simulink model "Experiment_134_cs"  (Simulink 10.1)
settings: Solver=ode8  StartTime=0.0  StopTime=20  FixedStep=1/10  RelTol=1e-3
model workspace (MAT data in the model file):
  mbox_table : struct (value not decoded)
  model_closed = 0
  sim_status = 0
PreLoadFcn:
  | mbxruntime.callbacks.PreLoadFcn(bdroot);
PostLoadFcn:
  | mbxruntime.callbacks.PostLoadFcn(bdroot);
InitFcn:
  | mbxruntime.callbacks.InitFcn(bdroot);
StartFcn:
  | mbxruntime.callbacks.StartFcn(bdroot);
StopFcn:
  | mbxruntime.callbacks.StopFcn(bdroot);
undefined symbols (not defined in the file or in its folder): acce_1, acce_2, acce_3, brake, steer, steer_1, steer_2, steer_3, t0_1, t0_2, t0_3, throttle, v_1, v_2, v_3, v_4
libraries: simulink x79, simulink_extras x12, PreScanSimulinkLibrary x8
(part 1 of 9)
CloseFcn:
  | mbxruntime.callbacks.CloseFcn(bdroot);
settings Model: Creator=PRESCAN  LastModifiedBy=Administrator
settings DataIOCC: LimitDataPoints=on  SignalLoggingSaveFormat=ModelDataLogs
settings OptimizationCC: ExpressionDepthLimit=2147483647  InitFltsAndDblsToZero=on
settings DebuggingCC: SaveWithParameterizedLinksMsg=none  SignalResolutionControl=TryResolveAllWithWarning  MultiTaskDSMMsg=warning  MultiTaskCondExecSysMsg=none  FcnCallInpInsideContextMsg=warning  StateNameClashWarn=warning
settings ModelReferenceCC: UpdateModelReferenceTargets=IfOutOfDate
settings SFSimCC: SimParseCustomCode=off
settings SFSimCC: SimCustomHeaderCode=|
  | #include "prescan.h"
  | #include "prescan_platform.h"
settings GRTTargetCC: TargetFcnLib=ansi_tfl_tmw.mat

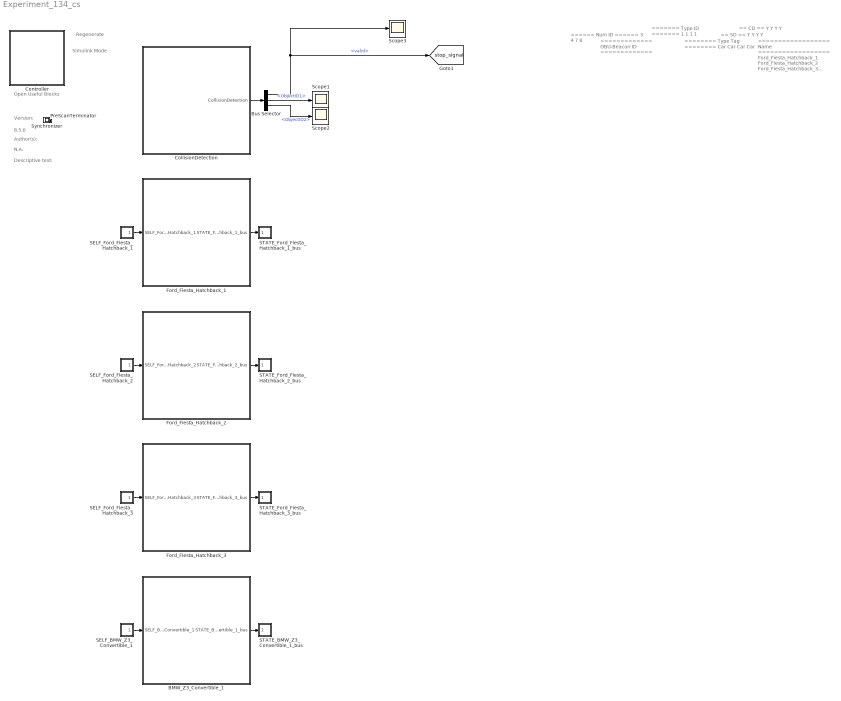
== system Experiment_134_cs ==
  note: Regenerate
  note: Simulink Mode
  note: Open Useful Blocks
  note: 8.5.0
  note: Version:
  note: Author(s):
  note: N.A.
  note: Descriptive text:
  note: ======
      | Num ID
      | ======
      | 3
      | 4
      | 7
      | 8
  note: =============
      | OBU-Beacon ID
      | =============
  note: =======
      | Type ID
      | =======
      | 1
      | 1
      | 1
      | 1
  note: ========
      | Type Tag
      | ========
      | Car
      | Car
      | Car
      | Car
  note: ==
      | SD
      | ==
      | Y
      | Y
      | Y
      | Y
  note: ==
      | CD
      | ==
      | Y
      | Y
      | Y
      | Y
  note: ==================
      | Name
      | ==================
      | Ford_Fiesta_Hatchback_1
      | Ford_Fiesta_Hatchback_2
      | Ford_Fiesta_Hatchback_3
      | BMW_Z3_Convertible_1
  BMW_Z3_Convertible_1 : Subsystem  Tag=WorldObjectSubSystem  InitFcn=UniqueId = '511';
      mask init:
      | modelPath = GenericModelHelper.getGenericModelFilePath('ModelDepo','Vehicles\BMW_Z3\BMW_Z3.pgmb','7699e47834166b94c09717861bab4f7a');imagePath = GenericModelHelper.getCompilationPicture(modelPath, 'BMW_Z3_HighPoly.png');
      mask Display: image(imread(imagePath));color('white');text(0, 0, ' ID=8\n')
  Bus Selector : BusSelector  OutputSignals=HEADER.valid,DATA.ObjectID1,DATA.ObjectID2
  CollisionDetection : Subsystem  Tag=sensor/CollisionDetection  Priority=1  LoadFcn=load('PrescanCollisionDetectionData.mat');load('PrescanCollisionDetectionMessage.mat')  mask(PreScan Source Block: CollisionDetection){}
      mask help: Collision Detection can be used to detect collisions between PreScan components. For Collision Detection the actual component shape is taken into account, so it is not a bounding box approach.
      settings: OpenFcn=open_system([gcb '/Sensor'],'mask')
      mask Help: eval('openHelp(811)')
      mask Display: image(imread('crash.jpg'))
  Controller : Subsystem  Description=648A510100055748DE7A0D51105FBAC79BDC343D1789F8D295123B632F6EF672  Priority=-1  LoadFcn=load PreScanControllerData  mask(PreScan Simulation Controller){prescanversion='8.5.0', ModelReferencing=off, TimeStep=1/10, ControlMode=0, PreScanExecutionMode=on, ControllerCount=0, ControllerIndex=0, ControllerOptions=''}
      mask prompts: prescanversion "PreScan Version"; ModelReferencing "Use Model Referencing"; TimeStep "Upload Period [s]"; ControlMode "Control Mode"; PreScanExecutionMode "Execution Mode"; ControllerCount "Controller Count"; ControllerIndex "Controller Index"; ControllerOptions "Controller Options"
      mask help:
      | Please do not remove this block from the compilation sheet,
      | as it connects the model to the PreScan environment.
      mask init:
      | model = bdroot(gcb);
      | ExperimentFile = mbxruntime.findExperimentFile(model,true); %relative path
      | 
      | [d1, d2, d3, prescandata] = prescan_Settings();
      | ModelDepo = fullfile(prescandata,'ModelDepo'); 
      | 
      | RTmode = mbxruntime.getRTMode(model);
      | 
      | SimulationMode = get_param(bdroot,'SimulationMode');
      | if strcmp(SimulationMode, 'rapid-accelerator')
      |     SimulationMode = 'external';
      | end
      | TargetName = get_param(bdroot,'SystemTargetFile');
      settings: ModelCloseFcn=assignin('base',['model_closed_' bdroot],true);
      mask Help: eval('openHelp(812)')
      mask Display: image(imread('prescanlogo.ico'))
  Ford_Fiesta_Hatchback_1 : Subsystem  Tag=WorldObjectSubSystem  InitFcn=UniqueId = '405';
      mask init:
      | modelPath = GenericModelHelper.getGenericModelFilePath('ModelDepo','Vehicles\Ford_Fiesta\Ford_Fiesta.pgmb','ee79ea2575daad9b4625620a37d79be4');imagePath = GenericModelHelper.getCompilationPicture(modelPath, 'Ford_Fiesta_HighPoly.png');
      mask Display: image(imread(imagePath));color('white');text(0, 0, ' ID=3\n')
  Ford_Fiesta_Hatchback_2 : Subsystem  Tag=WorldObjectSubSystem  InitFcn=UniqueId = '485';
      mask init: same as Experiment_134_cs/Ford_Fiesta_Hatchback_1
      mask Display: image(imread(imagePath));color('white');text(0, 0, ' ID=4\n')
  Ford_Fiesta_Hatchback_3 : Subsystem  Tag=WorldObjectSubSystem  InitFcn=UniqueId = '486';
      mask init: same as Experiment_134_cs/Ford_Fiesta_Hatchback_1
      mask Display: image(imread(imagePath));color('white');text(0, 0, ' ID=7\n')
  PreScanTerminator : Subsystem  Tag=PreScanTerminator  Priority=999  LoadFcn=load PrescanTerminatorData  mask(PreScan Simulation Terminator){TimeStep=1/10}
      mask prompts: TimeStep "Upload Period [s]"
      mask help:
      | Please do not remove this block from the compilation sheet as it
      | connects the model to the PreScan environment.
      mask Help: eval('openHelp(812)')
      mask Display: image(imread('prescanlogo.ico'))
  SELF_BMW_Z3_Convertible_1 : Subsystem  Tag=sensor/SelfPort  Priority=1  LoadFcn=load('PreScanSelfSensorData.mat')  mask(PreScan Source Block: SELF){}
      mask help:
      | The SELF port shows (state) information of the actor itself. The outputs are position in the experiment's axis system and the GPS coordinates, and the object's absolute velocity and compass heading.
      |
      | For more information, please click Help.
      settings: OpenFcn=open_system([gcb '/Sensor'],'mask')
      mask Help: eval('openHelp(462)')
      mask Display: image(imread('GPS.png'))
  SELF_Ford_Fiesta_Hatchback_1 : Subsystem  Tag=sensor/SelfPort  Priority=1  LoadFcn=load('PreScanSelfSensorData.mat')  mask(PreScan Source Block: SELF){}
      mask help:
      | The SELF port shows (state) information of the actor itself. The outputs are position in the experiment's axis system and the GPS coordinates, and the object's absolute velocity and compass heading.
      |
      | For more information, please click Help.
      settings: OpenFcn=open_system([gcb '/Sensor'],'mask')
      mask Help: eval('openHelp(462)')
      mask Display: image(imread('GPS.png'))
  SELF_Ford_Fiesta_Hatchback_2 : Subsystem  Tag=sensor/SelfPort  Priority=1  LoadFcn=load('PreScanSelfSensorData.mat')  mask(PreScan Source Block: SELF){}
      mask help:
      | The SELF port shows (state) information of the actor itself. The outputs are position in the experiment's axis system and the GPS coordinates, and the object's absolute velocity and compass heading.
      |
      | For more information, please click Help.
      settings: OpenFcn=open_system([gcb '/Sensor'],'mask')
      mask Help: eval('openHelp(462)')
      mask Display: image(imread('GPS.png'))
  SELF_Ford_Fiesta_Hatchback_3 : Subsystem  Tag=sensor/SelfPort  Priority=1  LoadFcn=load('PreScanSelfSensorData.mat')  mask(PreScan Source Block: SELF){}
      mask help:
      | The SELF port shows (state) information of the actor itself. The outputs are position in the experiment's axis system and the GPS coordinates, and the object's absolute velocity and compass heading.
      |
      | For more information, please click Help.
      settings: OpenFcn=open_system([gcb '/Sensor'],'mask')
      mask Help: eval('openHelp(462)')
      mask Display: image(imread('GPS.png'))
  STATE_BMW_Z3_Convertible_1_bus : Subsystem  Tag=actuator/StatePort  Priority=3  LoadFcn=load('PreScanStateActuatorData.mat')  mask(PreScan Sink Block: State){}
      mask help:
      | The Actor State contains a vector signal of size (9x1), containing the following signals:
      |
      | -  Position    	(x,y,z)             	[m]
      | -  Velocity    	(vx,vy,vz)         	[m/s]
      | -  Angles       	(Roll, Pitch, Yaw)	[rad]
      |
      | The Actor state is defined in the global axis system.
      | The state is superponed on the Initial position defined in the GUI.
      |
      | For more information, please click Help.
      settings: OpenFcn=open_system([gcb '/Actuator'],'mask')
      mask Help: eval('openHelp(222)')
      mask Display: image(imread('State.png'))
  STATE_Ford_Fiesta_Hatchback_1_bus : Subsystem  Tag=actuator/StatePort  Priority=3  LoadFcn=load('PreScanStateActuatorData.mat')  mask(PreScan Sink Block: State){}
      mask help:
      | The Actor State contains a vector signal of size (9x1), containing the following signals:
      |
      | -  Position    	(x,y,z)             	[m]
      | -  Velocity    	(vx,vy,vz)         	[m/s]
      | -  Angles       	(Roll, Pitch, Yaw)	[rad]
      |
      | The Actor state is defined in the global axis system.
      | The state is superponed on the Initial position defined in the GUI.
      |
      | For more information, please click Help.
      settings: OpenFcn=open_system([gcb '/Actuator'],'mask')
      mask Help: eval('openHelp(222)')
      mask Display: image(imread('State.png'))
  STATE_Ford_Fiesta_Hatchback_2_bus : Subsystem  Tag=actuator/StatePort  Priority=3  LoadFcn=load('PreScanStateActuatorData.mat')  mask(PreScan Sink Block: State){}
      mask help:
      | The Actor State contains a vector signal of size (9x1), containing the following signals:
      |
      | -  Position    	(x,y,z)             	[m]
      | -  Velocity    	(vx,vy,vz)         	[m/s]
      | -  Angles       	(Roll, Pitch, Yaw)	[rad]
      |
      | The Actor state is defined in the global axis system.
      | The state is superponed on the Initial position defined in the GUI.
      |
      | For more information, please click Help.
      settings: OpenFcn=open_system([gcb '/Actuator'],'mask')
      mask Help: eval('openHelp(222)')
      mask Display: image(imread('State.png'))
  STATE_Ford_Fiesta_Hatchback_3_bus : Subsystem  Tag=actuator/StatePort  Priority=3  LoadFcn=load('PreScanStateActuatorData.mat')  mask(PreScan Sink Block: State){}
      mask help:
      | The Actor State contains a vector signal of size (9x1), containing the following signals:
      |
      | -  Position    	(x,y,z)             	[m]
      | -  Velocity    	(vx,vy,vz)         	[m/s]
      | -  Angles       	(Roll, Pitch, Yaw)	[rad]
      |
      | The Actor state is defined in the global axis system.
      | The state is superponed on the Initial position defined in the GUI.
      |
      | For more information, please click Help.
      settings: OpenFcn=open_system([gcb '/Actuator'],'mask')
      mask Help: eval('openHelp(222)')
      mask Display: image(imread('State.png'))
  Scope1 : Scope
  Scope2 : Scope
  Scope3 : Scope
  Synchronizer : Subsystem  Tag=PreScanSynchronizer  Priority=2  LoadFcn=load PrescanSynchronizeData  mask(PreScan Simulation Core Block){TimeStep=1/10}
      mask prompts: TimeStep "Timestep [s]"
      mask help:
      | Please do not remove this block from the PreScan compilation sheet,
      | as it contains essential configuration parameters for a PreScan simulation.
      settings: DeleteFcn=PreScanBlockDeleteFcn;
      mask Display: image(imread('prescanlogo.ico'))
  tag scope: stop_signal=global
  wires:
  Bus Selector/3 -> Scope2/1  "<ObjectID2>"
  Bus Selector/2 -> Scope1/1  "<ObjectID1>"
  CollisionDetection/1(CollisionDetection) -> Bus Selector/1
  Bus Selector/1 -> Scope3/1, [stop_signal]  "<valid>"
  Ford_Fiesta_Hatchback_1/1(STATE_Ford_Fiesta_Hatchback_1_bus) -> STATE_Ford_Fiesta_Hatchback_1_bus/1(STATE_Ford_Fiesta_Hatchback_1_bus)
  SELF_Ford_Fiesta_Hatchback_1/1(SELF_Ford_Fiesta_Hatchback_1) -> Ford_Fiesta_Hatchback_1/1(SELF_Ford_Fiesta_Hatchback_1)
  Ford_Fiesta_Hatchback_2/1(STATE_Ford_Fiesta_Hatchback_2_bus) -> STATE_Ford_Fiesta_Hatchback_2_bus/1(STATE_Ford_Fiesta_Hatchback_2_bus)
  SELF_Ford_Fiesta_Hatchback_2/1(SELF_Ford_Fiesta_Hatchback_2) -> Ford_Fiesta_Hatchback_2/1(SELF_Ford_Fiesta_Hatchback_2)
  Ford_Fiesta_Hatchback_3/1(STATE_Ford_Fiesta_Hatchback_3_bus) -> STATE_Ford_Fiesta_Hatchback_3_bus/1(STATE_Ford_Fiesta_Hatchback_3_bus)
  SELF_Ford_Fiesta_Hatchback_3/1(SELF_Ford_Fiesta_Hatchback_3) -> Ford_Fiesta_Hatchback_3/1(SELF_Ford_Fiesta_Hatchback_3)
  BMW_Z3_Convertible_1/1(STATE_BMW_Z3_Convertible_1_bus) -> STATE_BMW_Z3_Convertible_1_bus/1(STATE_BMW_Z3_Convertible_1_bus)
  SELF_BMW_Z3_Convertible_1/1(SELF_BMW_Z3_Convertible_1) -> BMW_Z3_Convertible_1/1(SELF_BMW_Z3_Convertible_1)

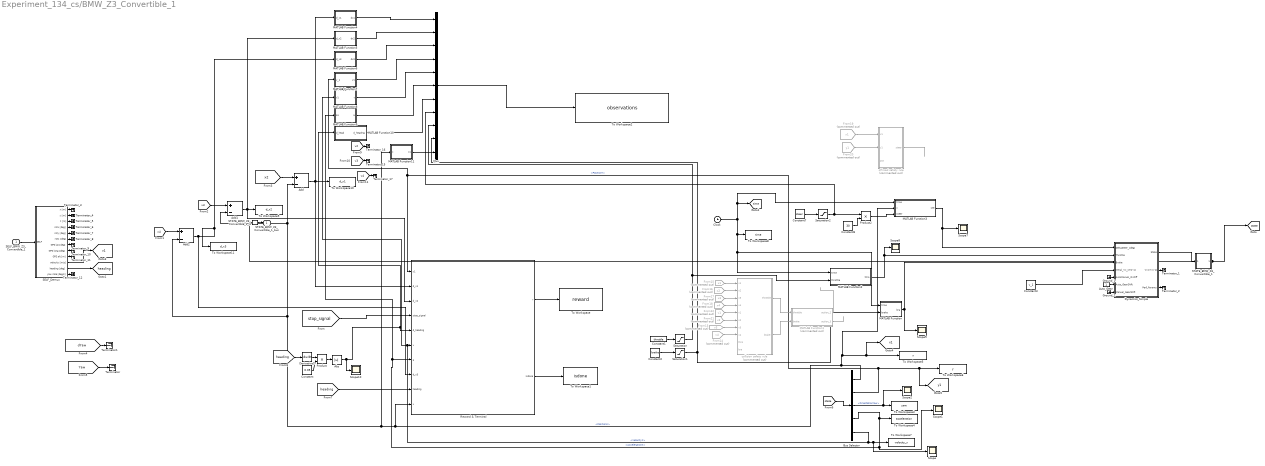
== system Experiment_134_cs/BMW_Z3_Convertible_1 ==
  SELF_BMW_Z3_Convertible_1 : Inport  Tag=inport/SelfPort  OutDataTypeStr=Bus: PRESCAN_SELFSENSORDATA  PortDimensions=1  SampleTime=1/10  BusOutputAsStruct=on
  Abs : Abs
  Add : Sum  Inputs=+-
  Add1 : Sum  Inputs=+-
  Add2 : Sum  Inputs=+-
  Auto_Gear : Constant  Tag=AutoGear
  Bus Selector : BusSelector  OutputSignals=PositionX,PositionY,OrientationYaw,AccelerationX,VelocityX
  Clock : Clock
  Constant : Constant  Value=0.05
  Constant1 : Constant  Value=throttle
  Constant2 : Constant  Value=brake
  Constant3 : Constant  Value=v_1
  Constant7 : Constant  Value=steer
  Constant8 : Constant  Value=30
  Derivative1 : Derivative
  Dynamics_Simple : Subsystem  Tag=Simple_Vehicle_Dynamics  mask(PreScan Block: Simple Dynamics){Migrate=on, TimeStep=1/10, ComputationMode=Continuous_Time}
      mask prompts: Migrate "Migrate. During migration this block will be replaced by a newer one."; TimeStep "Auto assigned: Time Step [s]"; ComputationMode "Computation mode:"
      mask help:
      | The Simple Dynamics Model is selected in the GUI to simulate vehicle dynamics behavior.
      |
      | The Simple Dynamics Model is completely open to the user. The parameters of this model can be set in the Simple Dynamics dialog in the GUI.
      |
      | For more information, please click Help.
      mask init:
      | p = SimpleDyn_pars;
      settings: DeleteFcn=PreScanBlockDeleteFcn;
      mask Help: eval('openHelp(220)')
      mask Display:
      | image(imread('SimpleDyn.png'))
      | port_label('input', 1, '{\delta}_S_t_ _e_e_r [deg]','texmode','on')
      | port_label('input', 2, 'Throttle [%]')
      | port_label('input', 3, 'Brake Pres [bar]')
      | port_label('input', 4, 'V_0 [ms-1]','texmode','on')
      | port_label('input', 5, 'Auto=[0]/Manual=[1]')
      | port_label('input', 6, 'Auto_GearShift')
      | port_label('input', 7, 'Manual_GearShift')
      | port_label('output', 1, 'State')
      | port_label('output', 2, 'Vx [ms-1]')
      | port_label('output', 3, 'Perf Params')
  From12 : From  Commented=on  GotoTag=v1  TagVisibility=global
  From13 : From  Commented=on  GotoTag=v3  TagVisibility=global
  From14 : From  Commented=on  GotoTag=v4  TagVisibility=global
  From15 : From  Commented=on  GotoTag=x1  TagVisibility=global
  From16 : From  Commented=on  GotoTag=x2  TagVisibility=global
  From17 : From  Commented=on  GotoTag=x3  TagVisibility=global
  From18 : From  Commented=on  GotoTag=x4  TagVisibility=global
  From19 : From  Commented=on  GotoTag=x1  TagVisibility=global
  From20 : From  Commented=on  GotoTag=y1  TagVisibility=global
  From21 : From  Commented=on  GotoTag=v2  TagVisibility=global
  Ground_1 : Ground
  Ground_2 : Ground
  MATLAB Function : MATLAB Function  TreatAsAtomicUnit=on
  MATLAB Function1 : MATLAB Function  Commented=on  TreatAsAtomicUnit=on
  MATLAB Function10 : MATLAB Function  TreatAsAtomicUnit=on
  MATLAB Function11 : MATLAB Function  TreatAsAtomicUnit=on
  MATLAB Function2 : MATLAB Function  TreatAsAtomicUnit=on
  MATLAB Function3 : MATLAB Function  TreatAsAtomicUnit=on
  MATLAB Function4 : MATLAB Function  TreatAsAtomicUnit=on
  MATLAB Function5 : MATLAB Function  TreatAsAtomicUnit=on
  MATLAB Function6 : MATLAB Function  TreatAsAtomicUnit=on
  MATLAB Function7 : MATLAB Function  TreatAsAtomicUnit=on
  MATLAB Function8 : MATLAB Function  TreatAsAtomicUnit=on
  MATLAB Function9 : MATLAB Function  TreatAsAtomicUnit=on
  Mux : Mux  Inputs=11
  Product : Product
  Product2 : Product
  Reward & Terminal : Subsystem
  SELF_Demux : Subsystem  Tag=demux/SelfPort  mask(PreScan Demux Block:){}
      mask help:
      | The SELF port shows (state) information of the actor itself. The outputs are position in the experiment's axis system and the GPS coordinates, and the object's absolute velocity and compass heading.
      |
      | For more information, please click Help.
      settings: DeleteFcn=PreScanBlockDeleteFcn;
      mask Help: eval('openHelp(462)')
      mask Display:
      | port_label('output',1,'x [m]')
      | port_label('output',2,'y [m]')
      | port_label('output',3,'z [m]','texmode','on')
      | port_label('output',4,'Rotx [deg]','texmode','on')
      | port_label('output',5,'Roty [deg]','texmode','on')
      | port_label('output',6,'Rotz [deg]','texmode','on')
      | port_label('output',7,'GPS lat [deg]','texmode','on')
      | port_label('output',8,'GPS long [deg]','texmode','on')
      | port_label('output',9,'GPS alt [m]','texmode','on')
      | port_label('output',10,'Velocity [m/s]')
      | port_label('output',11,'Heading [deg]')
      | port_label('output',12,'Yaw rate [deg/s]')
  STATE_BMW_Z3_Convertible_1 : Subsystem  Tag=mux/StatePort  Priority=0  LoadFcn=load PrescanStateActuatorData  mask(PreScan Sink Block: State){x0=-2.5, y0=3, z0=0.5, Roll0=0, Pitch0=0, Yaw0=0, TimeStep=1/10}
      mask prompts: x0 "Ini x-position VEHICLE wrt GLOBAL axis system [m]"; y0 "Ini y-position VEHICLE wrt GLOBAL axis system [m]"; z0 "Ini z-position VEHICLE wrt GLOBAL axis system [m]"; Roll0 "Ini roll-angle BODY wrt VEHICLE axis system [deg]"; Pitch0 "Ini pitch-angle BODY wrt VEHICLE axis system [deg]"; Yaw0 "Ini yaw-angle VEHICLE wrt GLOBAL axis system [deg]"; TimeStep "Auto-Assigned: Upload Period [s]"
      mask help:
      | The Actor State contains a vector signal of size (9x1), containing the following signals:
      |
      | -  Position                  (x,y,z)                                     [m]
      | -  Velocity                  (vx,vy,vz)                               [m/s]
      | -  Angles                    (Roll, Pitch, Yaw)                   [rad]
      |
      | The Actor state is defined in the global axis system.
      | The state is superponed on the Initial position defined in the GUI.
      |
      | For more information, please click Help.
      settings: DeleteFcn=PreScanBlockDeleteFcn;
      mask Help: eval('openHelp(222)')
      mask Display: image(imread('State.png'))
  STATE_BMW_Z3_Convertible_1_rc : RateTransition  Tag=mux_rc/StatePort  OutPortSampleTimeOpt=Inherit
  Saturation : Saturate  UpperLimit=1  LowerLimit=-1
  Saturation1 : Saturate  UpperLimit=1  LowerLimit=-1
  Saturation2 : Saturate  UpperLimit=1  LowerLimit=-1
  Scope{,1..2,7..10} (7 alike) : Scope
  Terminator : Terminator
  Terminator1 : Terminator
  Terminator_{1..12,15..17} (15 alike) : Terminator
  To Workspace : ToWorkspace  VariableName=reward  SampleTime=-1
      settings: MaxDataPoints=1  Save2DSignal=2-D array (concatenate along first dimension)
  To Workspace1 : ToWorkspace  VariableName=isdone  SampleTime=-1
      settings: MaxDataPoints=1  Save2DSignal=2-D array (concatenate along first dimension)
  To Workspace10 : ToWorkspace  VariableName=d_x1  SampleTime=-1
      settings: MaxDataPoints=1  Save2DSignal=2-D array (concatenate along first dimension)
  To Workspace11 : ToWorkspace  VariableName=d_x3  SampleTime=-1
      settings: MaxDataPoints=1  Save2DSignal=2-D array (concatenate along first dimension)
  To Workspace2 : ToWorkspace  VariableName=observations  SampleTime=-1
      settings: MaxDataPoints=1  Save2DSignal=2-D array (concatenate along first dimension)
  To Workspace3 : ToWorkspace  VariableName=yaw  SampleTime=-1
      settings: Save2DSignal=2-D array (concatenate along first dimension)
  To Workspace4 : ToWorkspace  VariableName=acceleration  SampleTime=-1
      settings: Save2DSignal=2-D array (concatenate along first dimension)
  To Workspace5 : ToWorkspace  VariableName=x  SampleTime=-1
      settings: Save2DSignal=2-D array (concatenate along first dimension)
  To Workspace6 : ToWorkspace  VariableName=y  SampleTime=-1
      settings: Save2DSignal=2-D array (concatenate along first dimension)
  To Workspace7 : ToWorkspace  VariableName=velocity_x  SampleTime=-1
      settings: Save2DSignal=2-D array (concatenate along first dimension)
  To Workspace8 : ToWorkspace  VariableName=time  SampleTime=-1
      settings: Save2DSignal=2-D array (concatenate along first dimension)
  To Workspace9 : ToWorkspace  VariableName=d_x2  SampleTime=-1
      settings: MaxDataPoints=1  Save2DSignal=2-D array (concatenate along first dimension)
  collision safety rule : Subsystem  Commented=on
  offroad safety rule : MATLAB Function  Commented=on  TreatAsAtomicUnit=on
  STATE_BMW_Z3_Convertible_1_bus : Outport  Tag=outport/StatePort  OutDataTypeStr=Bus: PRESCAN_STATEACTUATORDATA  PortDimensions=1  SampleTime=1/10
  tag scope: heading=global, state=global, time=global, v1=global, x1=global, y1=global
  wires:
  MATLAB Function3/1(ste) -> Dynamics_Simple/1(DeltaSteer_[deg]), Scope7/1
  MATLAB Function2/1(thro) -> Dynamics_Simple/2(Throttle), Scope8/1
  MATLAB Function/1(bra) -> Dynamics_Simple/3(Brake), Scope9/1
  Constant3/1 -> Dynamics_Simple/4(Initial_Vx_[ms-1])
  SELF_Demux/11(heading [deg]) -> [heading]
  MATLAB Function6/1(dx3) -> Mux/3
  [stop_signal] -> Reward & Terminal/4(stop_signal)
  [v4] -> Terminator_17/1
  Add1/1 -> MATLAB Function5/1(d_x2), Reward & Terminal/3(d_x2), To Workspace9/1
  [v2] -> Terminator_16/1
  Saturation1/1 -> MATLAB Function/2(brake), Mux/10
  Mux/1 -> To Workspace2/1
  Constant2/1 -> Saturation1/1
  Constant7/1 -> Saturation2/1
  [state] -> Bus Selector/1
  Bus Selector/3 -> Scope2/1, To Workspace3/1  "<OrientationYaw>"
  Bus Selector/4 -> MATLAB Function9/1(a1), Reward & Terminal/7(a), Scope1/1, To Workspace4/1  "<AccelerationX>"
  Bus Selector/1 -> Reward & Terminal/10(x), MATLAB Function11/1(x), Add1/2, Add/2, Add2/2, MATLAB Function3/2(x), [x1], To Workspace5/1  "<PositionX>"
  Reward & Terminal/2(isdone) -> To Workspace1/1
  MATLAB Function5/1(dx2) -> Mux/2
  [heading] -> Reward & Terminal/9(heading)
  MATLAB Function4/1(dx1) -> Mux/1
  [x4] -> Add2/1
  Product2/1 -> MATLAB Function3/3(steer)
  MATLAB Function1/2(action_3) -> ?
  Reward & Terminal/1(r) -> To Workspace/1
  MATLAB Function1/1(action_2) -> ?
  Constant1/1 -> Saturation/1
  Saturation/1 -> MATLAB Function2/2(throttle), Mux/9
  Add2/1 -> MATLAB Function6/1(d_x3), To Workspace11/1, Reward & Terminal/8(d_x3)
  Bus Selector/2 -> MATLAB Function7/1(y_1), Reward & Terminal/1(y1), [y1], To Workspace6/1  "<PositionY>"
  [x3] -> Add1/1
  MATLAB Function11/1(x1) -> Mux/11
  Constant8/1 -> Product2/2
  Bus Selector/5 -> MATLAB Function8/1(v1), Reward & Terminal/6(v), Scope/1, To Workspace7/1  "<VelocityX>"
  Add/1 -> MATLAB Function4/1(d_x1), Reward & Terminal/2(d_x1), To Workspace10/1
  Abs/1 -> MATLAB Function10/1(d_head), Reward & Terminal/5(d_heading), Scope10/1
  MATLAB Function7/1(y1) -> Mux/4
  MATLAB Function9/1(a) -> Mux/6
  [x2] -> Add/1
  MATLAB Function10/1(d_heading) -> Mux/7
  Saturation2/1 -> Mux/8, Product2/1
  Derivative1/1 -> Product/1
  Product/1 -> Abs/1
  [v3] -> Terminator_15/1
  Clock/1 -> MATLAB Function3/1(time), [time], MATLAB Function2/1(time), MATLAB Function/1(time), To Workspace8/1
  Constant/1 -> Product/2
  MATLAB Function8/1(v) -> Mux/5
  [heading] -> Derivative1/1
  STATE_BMW_Z3_Convertible_1/1(StateBus) -> [state], STATE_BMW_Z3_Convertible_1_rc/1
  [dYaw] -> Terminator1/1
  [Yaw] -> Terminator/1
  SELF_Demux/10(velocity [m/s]) -> [v1]
  collision safety rule/1(throttle) -> MATLAB Function1/1(throttle)
  collision safety rule/2(brake) -> MATLAB Function1/2(brake)
  From15/1 -> collision safety rule/1(x1)
  From16/1 -> collision safety rule/2(x2)
  From18/1 -> collision safety rule/4(x4)
  From17/1 -> collision safety rule/3(x3)
  From12/1 -> collision safety rule/5(v1)
  From21/1 -> collision safety rule/6(v2)
  From13/1 -> collision safety rule/7(v3)
  From14/1 -> collision safety rule/8(v4)
  offroad safety rule/1(steer) -> ?
  From19/1 -> offroad safety rule/1(x1)
  From20/1 -> offroad safety rule/2(y1)
  STATE_BMW_Z3_Convertible_1_rc/1 -> STATE_BMW_Z3_Convertible_1_bus/1
  SELF_BMW_Z3_Convertible_1/1 -> SELF_Demux/1(SELF)
  Auto_Gear/1 -> Dynamics_Simple/6(Auto_GearShift)
  Dynamics_Simple/1(State) -> STATE_BMW_Z3_Convertible_1/1(State)
  Ground_1/1 -> Dynamics_Simple/5(AutoManual_OnOff)
  Ground_2/1 -> Dynamics_Simple/7(Manual_GearShift)
  Dynamics_Simple/2(Vx [m s-1]) -> Terminator_1/1
  Dynamics_Simple/3(Perf_Params) -> Terminator_2/1
  SELF_Demux/1(x [m]) -> Terminator_3/1
  SELF_Demux/2(y [m]) -> Terminator_4/1
  SELF_Demux/3(z [m]) -> Terminator_5/1
  SELF_Demux/4(rotx [deg]) -> Terminator_6/1
  SELF_Demux/5(roty [deg]) -> Terminator_7/1
  SELF_Demux/6(rotz [deg]) -> Terminator_8/1
  SELF_Demux/7(GPS lat [deg]) -> Terminator_9/1
  SELF_Demux/8(GPS long [deg]) -> Terminator_10/1
  SELF_Demux/9(GPS alt [m]) -> Terminator_11/1
  SELF_Demux/12(yaw rate [deg/s]) -> Terminator_12/1

== system Experiment_134_cs/CollisionDetection ==
  Sensor : S-Function  FunctionName=sfun_CollisionDetection  Parameters=detectableCollisions, timestep  SFunctionDeploymentMode=off  EnableBusSupport=off  mask(PreScan Source Block: CollisionDetection){detectableCollisions=1, timestep=1/10}
      mask prompts: detectableCollisions "Max detectable collisions:"; timestep "MATLAB timestep:"
      mask help: Collision Detection can be used to detect collisions between PreScan components. For Collision Detection the actual component shape is taken into account, so it is not a bounding box approach.
      mask Help: eval('openHelp(811)')
      mask Display: image(imread('crash.jpg'))
  CollisionDetection : Outport  Tag=outport/CollisionDetection  OutDataTypeStr=Bus: PRESCAN_COLLISIONDETECTION_MESSAGE  PortDimensions=1  SampleTime=1/10
  wires:
  Sensor/1 -> CollisionDetection/1

== system Experiment_134_cs/Controller ==
  Terminator : Terminator
  sfun_Controller : S-Function  FunctionName=sfun_Controller  Parameters=SParameter1, SParameter2, SParameter3, SParameter4, SParameter5, SParameter6, SParameter7, SParameter8, SParameter9, SParameter10, SampleTime  SFunctionDeploymentMode=off  EnableBusSupport=off  mask(Legacy Function){SFunctionSpec=void prescan_outputFcn(void** work1, PRESCAN_CONTROLLERDATA y1[1]), SParameter1=uint8([ExperimentFile 0]), SParameter2=uint8([ModelDepo 0]), SParameter3=uint8([ControllerOptions 0]), SParameter4=RTmode, SParameter5=PreScanExecutionMode, SParameter6=ControlMode, SParameter7=ControllerCount, SParameter8=ControllerIndex, SParameter9=uint8([SimulationMode 0]), SParameter10=uint8([TargetName 0]), SampleTime=TimeStep, ShowSpec=on}
      mask prompts: SParameter1 "P1:"; SParameter2 "P2:"; SParameter3 "P3:"; SParameter4 "P4:"; SParameter5 "P5:"; SParameter6 "P6:"; SParameter7 "P7:"; SParameter8 "P8:"; SParameter9 "P9:"; SParameter10 "P10:"; SampleTime "Sample time (-1 for inherited):"; ShowSpec "Display function specification"
      mask help:
      | This block allows you to call the legacy functions specified by the following Legacy Code Tool definition:
      | def.SFunctionName = 'sfun_Controller';
      | def.OutputFcnSpec = 'void prescan_outputFcn(void** work1, PRESCAN_CONTROLLERDATA y1[1])';
      | def.StartFcnSpec = 'void prescan_startFcn(void ** work1, uint8 p1[], uint8 p2[], uint8 p3[], double p4, double p5, double p6, double p7, double p8, uint8 p9[], uint8 p10[])';
      | def.TerminateFcnSpec = 'void prescan_terminateFcn(void** work1)';
      | def.HeaderFiles = {'prescan_controller_data.h', 'prescan_SFunLibrary.h', 'prescan_CreateLogHandler.h', 'prescan_CreateErrorHandler.h', 'prescan_modify.h', 'ModuleDLL.h'};
      | def.SourceFiles = {'prescan_MexLogHandler.c', 'prescan_SimStructErrorHandler.c', 'prescan_LogHandler.c', 'prescan_ErrorHandler.c', 'prescan_Modify.c'};
      | def.HostLibFiles = {'sensorinterfaced.lib'};
      | def.TargetLibFiles = {'sensorinterfaced.so'};
      | def.IncPaths = {'.', 'C:\projects\prescan\rt_vislibrary\vis\..\pimp\include\sensors\InterfaceRTW'};
      | def.SrcPaths = {'C:\projects\prescan\rt_vislibrary\vis\..\pimp\include\sensors\InterfaceRTW', 'C:\projects\prescan\rt_vislibrary\vis\..\pimp\include\sensors\InterfaceRTW\ccurrt'};
      | def.LibPaths = {'C:\\projects\\prescan\\vislibrary_build\lib'};
      | def.SampleTime = 'parameterized';
      mask Help: <p>This block was generated automatically by the Legacy Code Tool. For detailed help on this tool, call<a href="matlab:legacy_code('help')"> legacy_code('help')</a>.</p>
      mask Callback ShowSpec:
      | if strcmp(get_param(gcbh, 'ShowSpec'), 'on')
      |   set_param(gcbh, 'MaskDisplay', sprintf('fprintf(''%s'');', get_param(gcbh, 'SFunctionSpec')));
      | else
      |   set_param(gcbh, 'MaskDisplay', sprintf('fprintf(''%s'');', get_param(gcbh, 'FunctionName')));
      | end
      mask Display: fprintf('void prescan_outputFcn(void** work1, PRESCAN_CONTROLLERDATA y1[1])');
  wires:
  sfun_Controller/1 -> Terminator/1

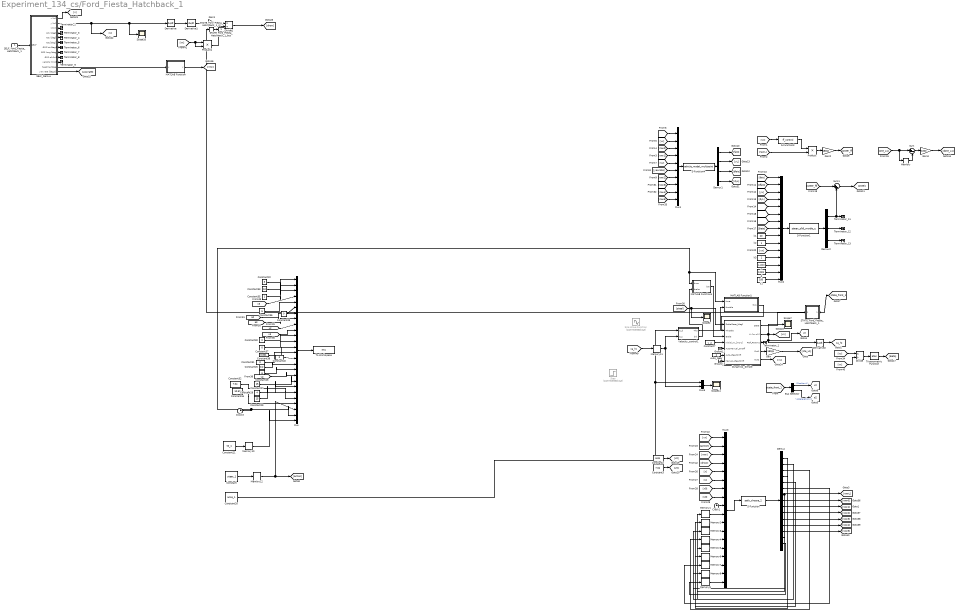
== system Experiment_134_cs/Ford_Fiesta_Hatchback_1 ==
  SELF_Ford_Fiesta_Hatchback_1 : Inport  Tag=inport/SelfPort  OutDataTypeStr=Bus: PRESCAN_SELFSENSORDATA  PortDimensions=1  SampleTime=1/10  BusOutputAsStruct=on
  Auto_Gear : Constant  Tag=AutoGear
  Bus Selector : BusSelector  OutputSignals=PositionX,AccelerationX
  Clock1 : Clock
  Clock3 : Clock
  Constant : Constant  Value=steer_1
  Constant2 : Constant  Value=6.81
  Constant20 : Constant  Value=acce_1
  Constant21 : Constant  Value=t0_1
  Constant22 : Constant  Value=3
  Constant25 : Constant  Value=0.2
  Constant26 : Constant  Value=6
  Constant27 : Constant  Value=15
  Constant28 : Constant  Value=4
  Constant29 : Constant  Value=15
  Constant3 : Constant  Value=7.04
  Constant{30..31,37,39..40} (5 alike) : Constant  Value=0
  Constant32 : Constant  Value=7.04
  Constant33 : Constant  Value=10
  Constant34 : Constant  Value=10.52
  Constant35 : Constant
  Constant36 : Constant  Value=5
  Constant38 : Constant  Value=0.001
  Constant7 : Constant  Value=v_2
  Demux : Demux  Outputs=15
  Demux1 : Demux
  Demux2 : Demux  Outputs=3
  Derivative : Derivative
  Derivative1 : Derivative
  Derivative2 : Derivative
  Divide : Product  Inputs=*/
  Divide1 : Product  Inputs=*/
  Dynamics_Simple : Subsystem  Tag=Simple_Vehicle_Dynamics  mask(PreScan Block: Simple Dynamics){Migrate=on, TimeStep=1/10, ComputationMode=Continuous_Time}
      mask prompts: Migrate "Migrate. During migration this block will be replaced by a newer one."; TimeStep "Auto assigned: Time Step [s]"; ComputationMode "Computation mode:"
      mask help:
      | The Simple Dynamics Model is selected in the GUI to simulate vehicle dynamics behavior.
      |
      | The Simple Dynamics Model is completely open to the user. The parameters of this model can be set in the Simple Dynamics dialog in the GUI.
      |
      | For more information, please click Help.
      mask init:
      | p = SimpleDyn_pars;
      settings: DeleteFcn=PreScanBlockDeleteFcn;
      mask Help: eval('openHelp(220)')
      mask Display:
      | image(imread('SimpleDyn.png'))
      | port_label('input', 1, '{\delta}_S_t_ _e_e_r [deg]','texmode','on')
      | port_label('input', 2, 'Throttle [%]')
      | port_label('input', 3, 'Brake Pres [bar]')
      | port_label('input', 4, 'V_0 [ms-1]','texmode','on')
      | port_label('input', 5, 'Auto=[0]/Manual=[1]')
      | port_label('input', 6, 'Auto_GearShift')
      | port_label('input', 7, 'Manual_GearShift')
      | port_label('output', 1, 'State')
      | port_label('output', 2, 'Vx [ms-1]')
      | port_label('output', 3, 'Perf Params')
  Gain : Gain  Gain=180/pi
  Gain1 : Gain
  Gain2 : Gain  Gain=180/pi
  Gain3 : Gain  Gain=1000
  Ground_1 : Ground
  Ground_2 : Ground
  MATLAB Function : MATLAB Function  TreatAsAtomicUnit=on
  MATLAB Function1 : MATLAB Function  TreatAsAtomicUnit=on
  MATLAB Function4 : MATLAB Function  TreatAsAtomicUnit=on
  Memory{,1..9,11} (11 alike) : Memory
  Memory10 : Memory  InitialCondition=-3
  Memory12 : Memory  InitialCondition=7.04
  Mux : Mux  Inputs=26
  Mux1 : Mux  Inputs=10
  Mux2 : Mux  Inputs=15
  Mux3 : Mux  Inputs=18
  Mux5 : Mux  Inputs=2
  Product : Product
  Product1 : Product
  S-Function : S-Function  FunctionName=path_choose_2  SFunctionDeploymentMode=off  EnableBusSupport=off
  S-Function1 : S-Function  FunctionName=steer_slid_mode_c  SFunctionDeploymentMode=off  EnableBusSupport=off
  S-Function3 : S-Function  FunctionName=ff_control  SFunctionDeploymentMode=off  EnableBusSupport=off
  S-Function4 : S-Function  FunctionName=vehicle_model_multipoint  SFunctionDeploymentMode=off  EnableBusSupport=off
  SELF_Demux : Subsystem  Tag=demux/SelfPort  mask(PreScan Demux Block:){}
      mask help:
      | The SELF port shows (state) information of the actor itself. The outputs are position in the experiment's axis system and the GPS coordinates, and the object's absolute velocity and compass heading.
      |
      | For more information, please click Help.
      settings: DeleteFcn=PreScanBlockDeleteFcn;
      mask Help: eval('openHelp(462)')
      mask Display:
      | port_label('output',1,'x [m]')
      | port_label('output',2,'y [m]')
      | port_label('output',3,'z [m]','texmode','on')
      | port_label('output',4,'Rotx [deg]','texmode','on')
      | port_label('output',5,'Roty [deg]','texmode','on')
      | port_label('output',6,'Rotz [deg]','texmode','on')
      | port_label('output',7,'GPS lat [deg]','texmode','on')
      | port_label('output',8,'GPS long [deg]','texmode','on')
      | port_label('output',9,'GPS alt [m]','texmode','on')
      | port_label('output',10,'Velocity [m/s]')
      | port_label('output',11,'Heading [deg]')
      | port_label('output',12,'Yaw rate [deg/s]')
  STATE_Ford_Fiesta_Hatchback_1 : Subsystem  Tag=mux/StatePort  Priority=0  LoadFcn=load PrescanStateActuatorData  mask(PreScan Sink Block: State){x0=-2.5, y0=7.04, z0=0.5, Roll0=0, Pitch0=0, Yaw0=0, TimeStep=1/10}
      mask prompts: x0 "Ini x-position VEHICLE wrt GLOBAL axis system [m]"; y0 "Ini y-position VEHICLE wrt GLOBAL axis system [m]"; z0 "Ini z-position VEHICLE wrt GLOBAL axis system [m]"; Roll0 "Ini roll-angle BODY wrt VEHICLE axis system [deg]"; Pitch0 "Ini pitch-angle BODY wrt VEHICLE axis system [deg]"; Yaw0 "Ini yaw-angle VEHICLE wrt GLOBAL axis system [deg]"; TimeStep "Auto-Assigned: Upload Period [s]"
      mask help:
      | The Actor State contains a vector signal of size (9x1), containing the following signals:
      |
      | -  Position                  (x,y,z)                                     [m]
      | -  Velocity                  (vx,vy,vz)                               [m/s]
      | -  Angles                    (Roll, Pitch, Yaw)                   [rad]
      |
      | The Actor state is defined in the global axis system.
      | The state is superponed on the Initial position defined in the GUI.
      |
      | For more information, please click Help.
      settings: DeleteFcn=PreScanBlockDeleteFcn;
      mask Help: eval('openHelp(222)')
      mask Display: image(imread('State.png'))
  STATE_Ford_Fiesta_Hatchback_1_rc : RateTransition  Tag=mux_rc/StatePort  OutPortSampleTimeOpt=Inherit
  Scope{2,7,10..11} (4 alike) : Scope
  Sine Wave Function : Sin  Commented=on  SampleTime=0
  Step : Step  Commented=on  Time=2  Before=7.04  After=10.52  SampleTime=0
  Sum : Sum  Inputs=|+-
  Sum1 : Sum  Inputs=|++
  Terminator_{1..9,11..13} (12 alike) : Terminator
  To Workspace : ToWorkspace  VariableName=IM1  SampleTime=-1
      settings: MaxDataPoints=1  Save2DSignal=2-D array (concatenate along first dimension)
  Trigonometric Function : Trigonometry  Operator=atan
  Velocity_control1 : Subsystem
  c : Constant  Value=14000
  c1 : Constant  Value=100
  d : Constant  Value=0.001
  k1 : Constant  Value=20
  k2 : Constant
  k3 : Constant
  STATE_Ford_Fiesta_Hatchback_1_bus : Outport  Tag=outport/StatePort  OutDataTypeStr=Bus: PRESCAN_STATEACTUATORDATA  PortDimensions=1  SampleTime=1/10
  tag scope: a2=global, state_front_1=global, v2=global, x2=global
  wires:
  [dste_L1] -> Mux2/6
  Constant2/1 -> [x0]
  [x0] -> Mux3/7
  [ste_L1] -> Mux2/5
  [yL] -> Mux2/3
  d/1 -> Mux2/14
  [raw5] -> Mux1/10
  [raw3] -> Mux1/8
  [y0] -> Mux3/8
  [steer_ff] -> Mux2/7
  Constant3/1 -> [y0]
  [vx] -> Mux2/11
  Sum/1 -> Gain3/1
  [faio] -> Mux2/1
  Gain3/1 -> [dste_L1]
  Mux1/1 -> S-Function4/1
  [vx] -> Mux3/1
  [dfaio] -> Mux2/2
  [x] -> Mux3/5
  Demux1/4 -> [dyL]
  [drow] -> Mux3/4
  [row] -> Mux3/3
  Mux3/1 -> S-Function/1
  Product/1 -> Gain2/1
  [rawL] -> Product/2
  Demux2/2 -> Terminator_12/1
  Demux1/2 -> [yL]
  c/1 -> Mux2/13
  [vx] -> S-Function3/1
  k2/1 -> Mux2/10
  Memory/1 -> Sum/2
  Demux2/1 -> Terminator_11/1, Sum1/2
  Demux2/3 -> Terminator_13/1
  c1/1 -> Mux2/15
  [Beta] -> Mux2/8
  Demux1/1 -> [faio]
  S-Function1/1 -> Demux2/1
  [steer_ff] -> Sum1/1
  [dyL] -> Mux2/4
  [yawrate] -> Mux1/6
  Mux2/1 -> S-Function1/1
  [vx] -> Mux1/2
  [vy] -> Mux1/5
  [raw1] -> Mux1/4
  [ste_L1] -> Mux1/1
  [ste_L1] -> Memory/1, Sum/1
  [raw0] -> Mux1/3
  Demux1/3 -> [dfaio]
  Dynamics_Simple/1(State) -> STATE_Ford_Fiesta_Hatchback_1/1(State)
  S-Function3/1 -> Product/1
  Sum1/1 -> [steel]
  k1/1 -> Mux2/9
  SELF_Demux/2(y [m]) -> [y], Scope10/1, Derivative/1
  [raw4] -> Mux1/9
  S-Function4/1 -> Demux1/1
  [raw2] -> Mux1/7
  S-Function/1 -> Demux/1
  k3/1 -> Mux2/12
  SELF_Demux/11(heading [deg]) -> MATLAB Function/1(u)
  [y] -> Mux3/6
  [action] -> Mux3/2
  Gain2/1 -> [steer_ff]
  Constant7/1 -> Dynamics_Simple/4(Initial_Vx_[ms-1])
  Dynamics_Simple/4(Out1) -> Gain/1
  Gain/1 -> [ste_L1]
  [steel] -> Dynamics_Simple/1(DeltaSteer_[deg]), Scope2/1
  Dynamics_Simple/2(Vx [m s-1]) -> Derivative2/1, [v2], Scope7/1, [vx]
  Demux/1 -> Memory2/1
  Demux/2 -> Memory3/1
  Demux/3 -> Memory4/1
  Demux/4 -> Memory5/1
  Demux/5 -> Memory6/1
  Demux/6 -> Memory7/1
  Demux/7 -> [rawL], Memory1/1
  Clock1/1 -> Mux3/9
  Memory1/1 -> Mux3/10
  Memory2/1 -> Mux3/11
  Memory3/1 -> Mux3/12
  Memory5/1 -> Mux3/14
  Memory6/1 -> Mux3/15
  Memory7/1 -> Mux3/16
  Memory4/1 -> Mux3/13
  Dynamics_Simple/5(Out2) -> [vy]
  [vy] -> Divide/1
  [vx] -> Divide/2
  Divide/1 -> Trigonometric Function/1
  Trigonometric Function/1 -> [Beta]
  MATLAB Function/1(y) -> [row]
  Derivative/1 -> Derivative1/1
  Derivative1/1 -> Gain1/1
  [vx] -> Product1/2, Product1/1
  Product1/1 -> Divide1/2
  Divide1/1 -> [drow]
  Gain1/1 -> Divide1/1
  Demux/8 -> [raw0]
  Demux/9 -> [raw1]
  Demux/10 -> [raw2]
  Demux/11 -> [raw3]
  Demux/13 -> [raw5]
  Demux/12 -> [raw4]
  Memory8/1 -> Mux3/17
  Demux/14 -> Memory8/1
  Memory9/1 -> Mux3/18
  Demux/15 -> Memory9/1
  Derivative2/1 -> [a_h]
  Mux5/1 -> Scope11/1
  Memory11/1 -> Mux5/2, Velocity_control1/2(a_t)
  SELF_Demux/1(x [m]) -> [x]
  SELF_Demux/12(yaw rate [deg/s]) -> [yawrate]
  STATE_Ford_Fiesta_Hatchback_1/1(StateBus) -> [state_front_1], STATE_Ford_Fiesta_Hatchback_1_rc/1
  Velocity_control1/1(Tho) -> MATLAB Function1/2(throttle)
  Velocity_control1/2(brk) -> MATLAB Function4/2(brake)
  [state_front_1] -> Bus Selector/1
  Bus Selector/2 -> [a2]  "<AccelerationX>"
  Bus Selector/1 -> [x2]  "<PositionX>"
  [a_h] -> Memory11/1
  MATLAB Function4/1(bra) -> Dynamics_Simple/3(Brake)
  MATLAB Function1/1(thro) -> Dynamics_Simple/2(Throttle)
  Constant20/1 -> Velocity_control1/1(a_d), Mux5/1
  Clock3/1 -> Mux/25, MATLAB Function1/1(time), MATLAB Function4/1(time)
  Mux/1 -> To Workspace/1
  Memory12/1 -> [action], Mux/24
  Constant/1 -> Memory12/1
  Memory10/1 -> Mux/26
  Constant21/1 -> Memory10/1
  [a2] -> Mux/7
  Constant22/1 -> Mux/1
  [a3] -> Mux/8
  Constant36/1 -> Mux/5
  Constant35/1 -> Mux/3
  [v3] -> Mux/4
  Constant33/1 -> Mux/2
  Constant39/1 -> Mux/6
  [x3] -> Mux/10
  [x2] -> Mux/9
  Constant30/1 -> Mux/11
  Constant37/1 -> Mux/12
  Constant38/1 -> Mux/13
  Constant31/1 -> Mux/14
  Constant40/1 -> Mux/15
  Constant25/1 -> Mux/16
  Constant26/1 -> Mux/17
  [v2] -> Mux/18
  Constant27/1 -> Mux/19
  Constant28/1 -> Mux/20
  Constant29/1 -> Mux/21
  Constant32/1 -> Mux/22
  Constant34/1 -> Mux/23
  STATE_Ford_Fiesta_Hatchback_1_rc/1 -> STATE_Ford_Fiesta_Hatchback_1_bus/1
  SELF_Ford_Fiesta_Hatchback_1/1 -> SELF_Demux/1(SELF)
  Auto_Gear/1 -> Dynamics_Simple/6(Auto_GearShift)
  Ground_1/1 -> Dynamics_Simple/5(AutoManual_OnOff)
  Ground_2/1 -> Dynamics_Simple/7(Manual_GearShift)
  Dynamics_Simple/3(Perf_Params) -> Terminator_1/1
  SELF_Demux/3(z [m]) -> Terminator_2/1
  SELF_Demux/4(rotx [deg]) -> Terminator_3/1
  SELF_Demux/5(roty [deg]) -> Terminator_4/1
  SELF_Demux/6(rotz [deg]) -> Terminator_5/1
  SELF_Demux/7(GPS lat [deg]) -> Terminator_6/1
  SELF_Demux/8(GPS long [deg]) -> Terminator_7/1
  SELF_Demux/9(GPS alt [m]) -> Terminator_8/1
  SELF_Demux/10(velocity [m/s]) -> Terminator_9/1
